simulink model "ss_robust_estimator_ADV"  (R2022b)
settings: Solver=VariableStepAuto  StartTime=0.0  StopTime=10.0  RelTol=1e-3
values from neighbouring files (symbols this model uses):
  degs2rpm = 0.166666666667    [parameters.mat]
  der =     [parameters.mat]
  rpm2rads = 0.10471975512    [parameters.mat]
  sens =     [parameters.mat]
  simul =     [parameters.mat]
  ssNominal =     [parameters.mat]
  ssRobust =     [parameters.mat]
  Ts = 0.001    [parameters.mat]
undefined symbols (not defined in the file or in its folder): DiscIntNeverNeededParam, redObs, T
settings Model: Creator=emanuelevitetta  LastModifiedBy=david

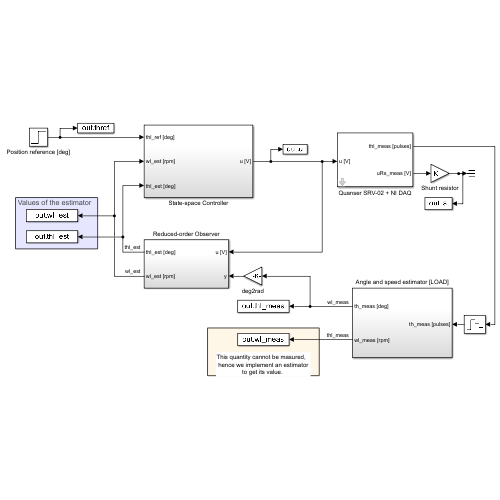
[thumbnail: Simulink's stored preview of the top-level diagram]
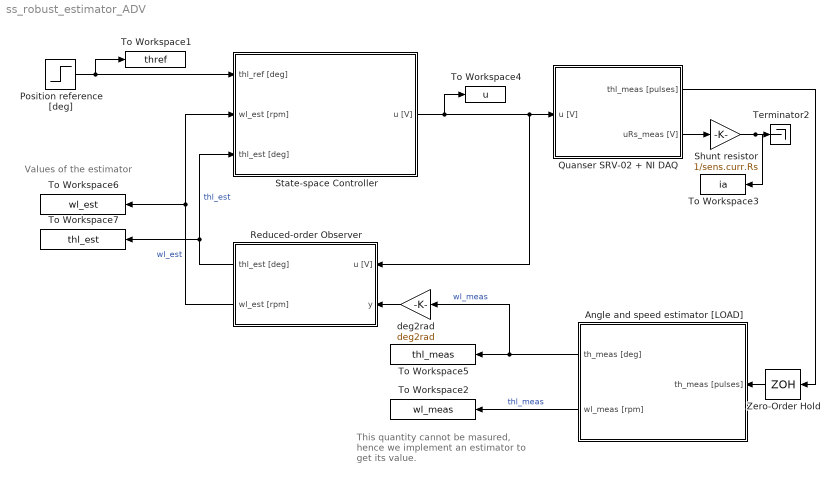
== system ss_robust_estimator_ADV ==
  note: This quantity cannot be masured,
      | hence we implement an estimator
      | to get its value.
  note: Values of the estimator
  Angle and speed estimator [LOAD] : Subsystem
  Position reference [deg] : Step  After=simul.stepdeg
  Quanser SRV-02 + NI DAQ : Subsystem  mask(Quanser SRV-02 (with inertial load) + NI DAQ){Ts=0.001, fricType=Coulomb + viscous}
      mask prompts: Ts "NI DAQ Sample Time:"; fricType "Friction model"
      mask help: Quanser SRV-02 (with inertial load) + NI DAQ model.
      mask init:
      | %%  Sensors data
      | 
      | %   shunt resistor
      | sens.curr.Rs = 0.5;                         %   resistance [Ohm]   
      | sens.curr.uRs_std = 0.01;                   %   voltage noise standard dev [V]                           
      | sens.curr.uRs_var = sens.curr.uRs_std^2;	%   voltage noise variance [V^2]
      | 
      | %   Hewlett-Packard HEDS-5540#A06 optical encoder
      | sens.enc.ppr = 500*4;                       %   pulses per rotation
      | sens.enc.pulse2deg = 360/sens.enc.ppr;      %   [pulses] -> [deg]
      | sens.enc.pulse2rad = 2*pi/sens.enc.ppr;     %   [pulses] -> [rad]
      | sens.enc.deg2pulse = sens.enc.ppr/360;      %   [deg] -> [pulses]
      | sens.enc.rad2pulse = sens.enc.ppr/2/pi;     %   [rad] -> [pulses]
      | 
      | 
      | %%  Data acquisition board (daq) data
      | 
      | %   NI PCI-6221 DAC data
      | daq.dac.bits = 16;                                  %   resolution (bits)
      | daq.dac.fs   = 10;                                  %   full scale 
      | daq.dac.q    = 2*daq.dac.fs/(2^daq.dac.bits-1);     %	quantization
      | 
      | %   NI PCI-6221 ADC data
      | daq.adc.bits = 16;                                  %   resolution (bits)
      | daq.adc.fs   = 10;                                  %   full scale (as set in SLDRT Analog Input block)
      | daq.adc.q    = 2*daq.adc.fs/(2^daq.adc.bits-1);     %   quantization
      mask Help:
      | Riccardo Antonello (antonello@dei.unipd.it)
      | 
      | April 24, 2020
      | 
      | Dept. of Information Engineering, University of Padova
      mask TypeOptions fricType: Coulomb + viscous | Karnopp
  Reduced-order Observer : Subsystem
  Shunt resistor : Gain  Gain=1/sens.curr.Rs
  State-space Controller : Subsystem
  Terminator2 : Terminator
  To Workspace1 : ToWorkspace  VariableName=thref  SaveFormat=Structure With Time  SampleTime=Ts
  To Workspace2 : ToWorkspace  VariableName=wl_meas  SaveFormat=Structure With Time  SampleTime=Ts
  To Workspace3 : ToWorkspace  VariableName=ia  SaveFormat=Structure With Time  SampleTime=Ts
  To Workspace4 : ToWorkspace  VariableName=u  SaveFormat=Structure With Time  SampleTime=Ts
  To Workspace5 : ToWorkspace  VariableName=thl_meas  SaveFormat=Structure With Time  SampleTime=Ts
  To Workspace6 : ToWorkspace  VariableName=wl_est  SaveFormat=Structure With Time  SampleTime=Ts
  To Workspace7 : ToWorkspace  VariableName=thl_est  SaveFormat=Structure With Time  SampleTime=Ts
  Zero-Order Hold : ZeroOrderHold  SampleTime=T(simul.Ts_selector)
  deg2rad : Gain  Gain=deg2rad
  wires:
  Quanser SRV-02 + NI DAQ/2(uRs_meas [V]) -> Shunt resistor/1
  Shunt resistor/1 -> To Workspace3/1, Terminator2/1
  Quanser SRV-02 + NI DAQ/1(thl_meas [pulses]) -> Zero-Order Hold/1
  Position reference [deg]/1 -> To Workspace1/1, State-space Controller/1(thl_ref [deg])
  Reduced-order Observer/2(wl_est [rpm]) -> To Workspace6/1, State-space Controller/2(wl_est [rpm])  "wl_est"
  State-space Controller/1(u [V]) -> To Workspace4/1, Reduced-order Observer/1(u [V]), Quanser SRV-02 + NI DAQ/1(u [V])
  Reduced-order Observer/1(thl_est [deg]) -> State-space Controller/3(thl_est [deg]), To Workspace7/1  "thl_est"
  deg2rad/1 -> Reduced-order Observer/2(y)
  Angle and speed estimator [LOAD]/1(th_meas [deg]) -> deg2rad/1, To Workspace5/1  "wl_meas"
  Angle and speed estimator [LOAD]/2(wl_meas [rpm]) -> To Workspace2/1  "thl_meas"
  Zero-Order Hold/1 -> Angle and speed estimator [LOAD]/1(th_meas [pulses])

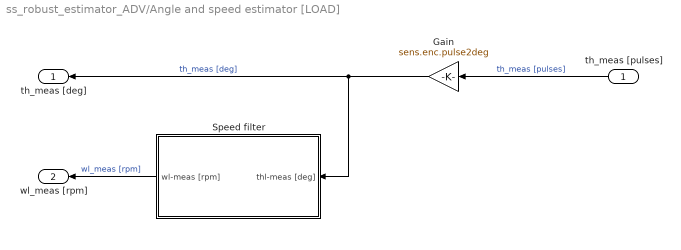
== system ss_robust_estimator_ADV/Angle and speed estimator [LOAD] ==
  th_meas [pulses] : Inport
  Gain : Gain  Gain=sens.enc.pulse2deg
  Speed filter : Subsystem
  th_meas [deg] : Outport
  wl_meas [rpm] : Outport  Port=2
  wires:
  Speed filter/1(wl-meas [rpm]) -> wl_meas [rpm]/1  "wl_meas [rpm]"
  th_meas [pulses]/1 -> Gain/1  "th_meas [pulses]"
  Gain/1 -> Speed filter/1(thl-meas [deg]), th_meas [deg]/1  "th_meas [deg]"

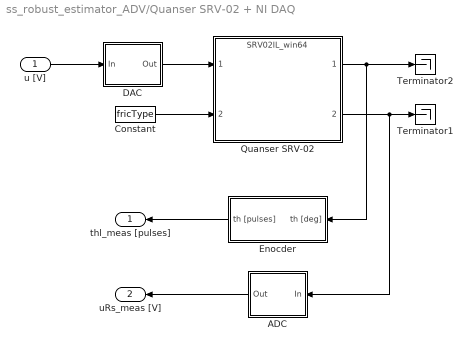
== system ss_robust_estimator_ADV/Quanser SRV-02 + NI DAQ ==
  u [V] : Inport
  ADC : Subsystem
  Constant : Constant  Value=fricType
  DAC : Subsystem
  Enocder : Subsystem
  Quanser SRV-02 : ModelReference  ModelNameDialog=SRV02IL_win64.slxp  ModelReferenceVersion=1.44  CopyOfModelProtected=on
  Terminator1 : Terminator
  Terminator2 : Terminator
  thl_meas [pulses] : Outport
  uRs_meas [V] : Outport  Port=2
  wires:
  Enocder/1(th [pulses]) -> thl_meas [pulses]/1
  ADC/1(Out) -> uRs_meas [V]/1
  DAC/1(Out) -> Quanser SRV-02/1
  Quanser SRV-02/2 -> ADC/1(In), Terminator1/1
  u [V]/1 -> DAC/1(In)
  Quanser SRV-02/1 -> Enocder/1(th [deg]), Terminator2/1
  Constant/1 -> Quanser SRV-02/2

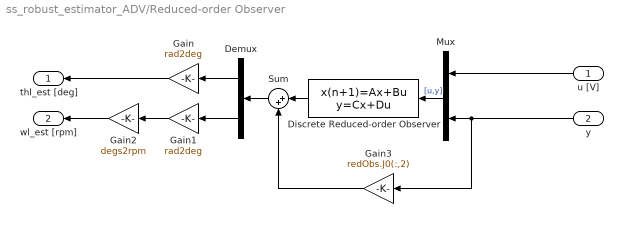
== system ss_robust_estimator_ADV/Reduced-order Observer ==
  u [V] : Inport
  y : Inport  Port=2
  Demux : Demux  Outputs=2
  Discrete Reduced-order Observer : DiscreteStateSpace  A=redObs.Ph0  B=redObs.Gamma0  C=redObs.H0  D=zeros(2)  SampleTime=T(simul.Ts_selector)
  Gain : Gain  Gain=rad2deg
  Gain1 : Gain  Gain=rad2deg
  Gain2 : Gain  Gain=degs2rpm
  Gain3 : Gain  Gain=redObs.J0(:,2)
  Mux : Mux  Inputs=2
  Sum : Sum  Inputs=|++
  thl_est [deg] : Outport
  wl_est [rpm] : Outport  Port=2
  wires:
  Demux/1 -> Gain/1
  Mux/1 -> Discrete Reduced-order Observer/1  "[u,y]"
  Demux/2 -> Gain1/1
  u [V]/1 -> Mux/1
  Gain/1 -> thl_est [deg]/1
  Gain1/1 -> Gain2/1
  Gain2/1 -> wl_est [rpm]/1
  y/1 -> Gain3/1, Mux/2
  Sum/1 -> Demux/1
  Discrete Reduced-order Observer/1 -> Sum/1
  Gain3/1 -> Sum/2

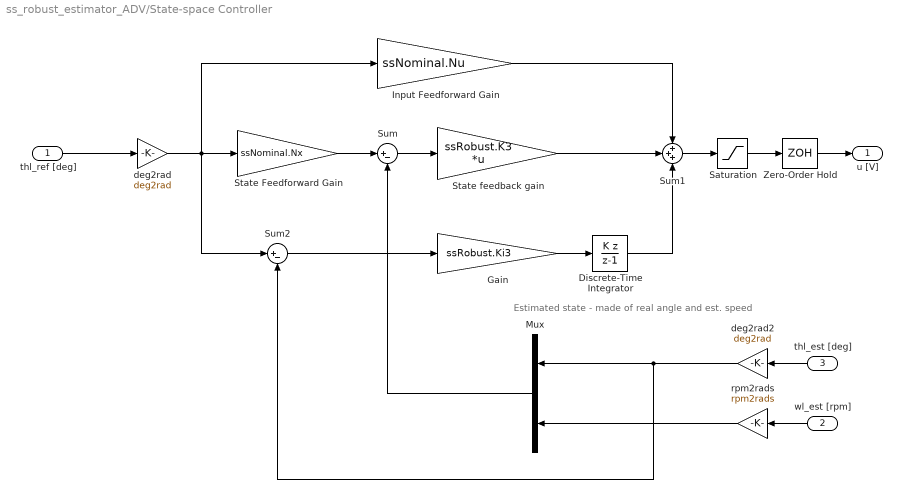
== system ss_robust_estimator_ADV/State-space Controller ==
  note: Estimated state - made of real angle and est. speed
  thl_ref [deg] : Inport
  wl_est [rpm] : Inport  Port=2
  thl_est [deg] : Inport  Port=3
  Discrete-Time Integrator : DiscreteIntegrator  IntegratorMethod=Accumulation: Backward Euler  SampleTime=T(simul.Ts_selector)  ICPrevOutput=DiscIntNeverNeededParam  ICPrevScaledInput=DiscIntNeverNeededParam
  Gain : Gain  Gain=ssRobust.Ki3
  Input Feedforward Gain : Gain  Gain=ssNominal.Nu
  Mux : Mux  Inputs=2
  Saturation : Saturate  UpperLimit=10  LowerLimit=-10
  State Feedforward Gain : Gain  Gain=ssNominal.Nx
  State feedback gain : Gain  Gain=ssRobust.K3  Multiplication=Matrix(K*u)
  Sum : Sum  Inputs=|+-
  Sum1 : Sum  Inputs=+++
  Sum2 : Sum  Inputs=|+-
  Zero-Order Hold : ZeroOrderHold  SampleTime=T(simul.Ts_selector)
  deg2rad : Gain  Gain=deg2rad
  deg2rad2 : Gain  Gain=deg2rad
  rpm2rads : Gain  Gain=rpm2rads
  u [V] : Outport
  wires:
  thl_est [deg]/1 -> deg2rad2/1
  wl_est [rpm]/1 -> rpm2rads/1
  Mux/1 -> Sum/2
  thl_ref [deg]/1 -> deg2rad/1
  deg2rad/1 -> Sum2/1, State Feedforward Gain/1, Input Feedforward Gain/1
  State Feedforward Gain/1 -> Sum/1
  Sum/1 -> State feedback gain/1
  State feedback gain/1 -> Sum1/2
  Sum1/1 -> Saturation/1
  Input Feedforward Gain/1 -> Sum1/1
  Gain/1 -> Discrete-Time Integrator/1
  Discrete-Time Integrator/1 -> Sum1/3
  Sum2/1 -> Gain/1
  deg2rad2/1 -> Mux/1, Sum2/2
  rpm2rads/1 -> Mux/2
  Saturation/1 -> Zero-Order Hold/1
  Zero-Order Hold/1 -> u [V]/1

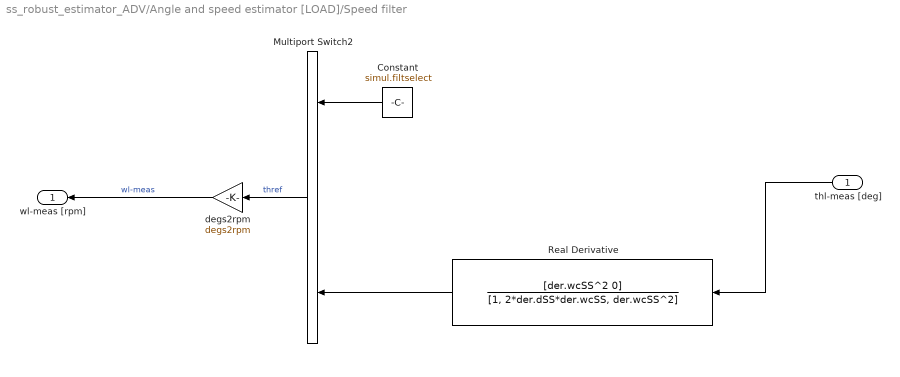
== system ss_robust_estimator_ADV/Angle and speed estimator [LOAD]/Speed filter ==
  thl-meas [deg] : Inport
  Constant : Constant  Value=simul.filtselect
  Multiport Switch2 : MultiPortSwitch  Inputs=2  SaturateOnIntegerOverflow=off  InputSameDT=off
  Real Derivative : TransferFcn  Numerator=[der.wcSS^2 0]  Denominator=[1, 2*der.dSS*der.wcSS, der.wcSS^2]
  degs2rpm : Gain  Gain=degs2rpm
  wl-meas [rpm] : Outport
  wires:
  degs2rpm/1 -> wl-meas [rpm]/1  "wl-meas"
  Real Derivative/1 -> Multiport Switch2/3
  Multiport Switch2/1 -> degs2rpm/1  "thref"
  Constant/1 -> Multiport Switch2/1
  thl-meas [deg]/1 -> Real Derivative/1

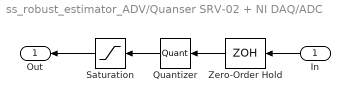
== system ss_robust_estimator_ADV/Quanser SRV-02 + NI DAQ/ADC ==
  In : Inport
  Quantizer : Quantizer  QuantizationInterval=daq.adc.q
  Saturation : Saturate  UpperLimit=daq.adc.fs  LowerLimit=-daq.adc.fs
  Zero-Order Hold : ZeroOrderHold  SampleTime=Ts
  Out : Outport
  wires:
  Saturation/1 -> Out/1
  In/1 -> Zero-Order Hold/1
  Quantizer/1 -> Saturation/1
  Zero-Order Hold/1 -> Quantizer/1

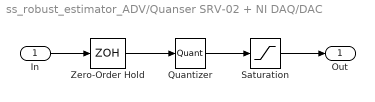
== system ss_robust_estimator_ADV/Quanser SRV-02 + NI DAQ/DAC ==
  In : Inport
  Quantizer : Quantizer  QuantizationInterval=daq.dac.q
  Saturation : Saturate  UpperLimit=daq.dac.fs  LowerLimit=-daq.dac.fs
  Zero-Order Hold : ZeroOrderHold  SampleTime=Ts
  Out : Outport
  wires:
  Quantizer/1 -> Saturation/1
  In/1 -> Zero-Order Hold/1
  Zero-Order Hold/1 -> Quantizer/1
  Saturation/1 -> Out/1

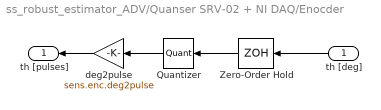
== system ss_robust_estimator_ADV/Quanser SRV-02 + NI DAQ/Enocder ==
  th [deg] : Inport
  Quantizer : Quantizer  QuantizationInterval=sens.enc.pulse2deg
  Zero-Order Hold : ZeroOrderHold  SampleTime=Ts
  deg2pulse : Gain  Gain=sens.enc.deg2pulse
  th [pulses] : Outport
  wires:
  Quantizer/1 -> deg2pulse/1
  th [deg]/1 -> Zero-Order Hold/1
  Zero-Order Hold/1 -> Quantizer/1
  deg2pulse/1 -> th [pulses]/1
